simulink model "hybrid_new_eq_circuit_pascal5_single_shot_stack"  (R2019a)
settings: Solver=FixedStepAuto  StartTime=0.0  StopTime=sim_time  FixedStep=resolution  MinStep=0.001  RelTol=1e-4  EnableMultiTasking=on
values from neighbouring files (symbols this model uses):
  amps_in = double(amps_in)    [ClassHybrid.m]    (also in Sc.m = double(amps_in_); workspace_test_model.mat = 0)
  resolution = double(resolution)    [ClassHybrid.m]    (also in Sc.m = double(resolution_); matlab.mat = 1; model_out_all.mat = 0.5; testHyb.m = 0.5)
  tStep = resolution    (= 0.1)    [ClassHybrid.m]    (also in Sc.m; matlab.mat = 10; model_out_all.mat = 1; raw.mat = 1)
libraries: powerlib x525, simulink x9
(part 3 of 8)

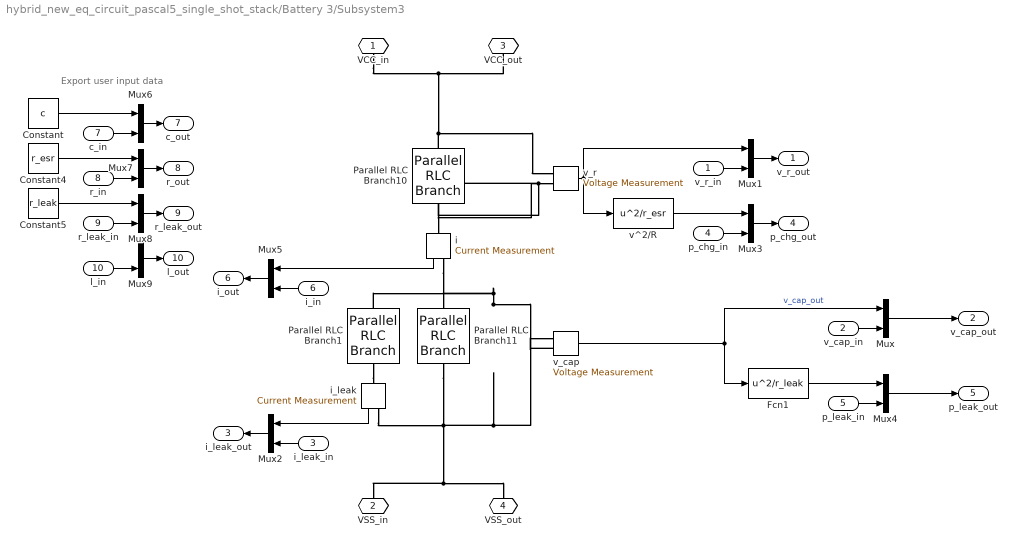
== system hybrid_new_eq_circuit_pascal5_single_shot_stack/Battery 3/Subsystem3 ==
  note: Export user input data
  v_r_in : Inport
  v_cap_in : Inport  Port=2
  i_leak_in : Inport  Port=3
  p_chg_in : Inport  Port=4
  p_leak_in : Inport  Port=5
  i_in : Inport  Port=6
  c_in : Inport  Port=7
  r_in : Inport  Port=8
  r_leak_in : Inport  Port=9
  l_in : Inport  Port=10
  Constant : Constant  Value=c
  Constant4 : Constant  Value=r_esr
  Constant5 : Constant  Value=r_leak
  Fcn1 : Fcn  Expr=u^2/r_leak
  Mux{,1..9} (10 alike) : Mux  Inputs=2
  Parallel RLC Branch1 : powerlib/Elements/Parallel RLC Branch  LConnTagsString=a  RConnTagsString=__new0  BranchType=R  Resistance=r_esr  Inductance=1e-3  SetiL0=off  InitialCurrent=0  Capacitance=1e-6  Setx0=off  InitialVoltage=0  Measurements=None
      settings: SourceProductName=Simscape Electrical
  Parallel RLC Branch10 : powerlib/Elements/Parallel RLC Branch  LConnTagsString=a  RConnTagsString=__new0  BranchType=R  Resistance=0.000001  Inductance=1e-3  SetiL0=off  InitialCurrent=0  Capacitance=1e-6  Setx0=off  InitialVoltage=0  Measurements=None
      settings: SourceProductName=Simscape Electrical
  Parallel RLC Branch11 : powerlib/Elements/Parallel RLC Branch  LConnTagsString=a  RConnTagsString=__new0  BranchType=C  Resistance=1  Inductance=1e-3  SetiL0=off  InitialCurrent=0  Capacitance=c  Setx0=on  InitialVoltage=v_init  Measurements=None
      settings: SourceProductName=Simscape Electrical
  i : powerlib/Measurements/Current Measurement  PhasorSimulation=off  OutputType=Complex  PSBequivalent=0
      settings: SourceProductName=Simscape Electrical
  i_leak : powerlib/Measurements/Current Measurement  PhasorSimulation=off  OutputType=Complex  PSBequivalent=0
      settings: SourceProductName=Simscape Electrical
  v^2/R : Fcn  Expr=u^2/r_esr
  v_cap : powerlib/Measurements/Voltage Measurement  PhasorSimulation=off  OutputType=Magnitude  PSBequivalent=0
      settings: SourceProductName=Simscape Electrical
  v_r : powerlib/Measurements/Voltage Measurement  PhasorSimulation=off  OutputType=Complex  PSBequivalent=0
      settings: SourceProductName=Simscape Electrical
  VCC_in : PMIOPort  Side=Left
  VSS_in : PMIOPort  Port=2  Side=Left
  VCC_out : PMIOPort  Tag=PMCPort  Port=3  Side=Right
  VSS_out : PMIOPort  Tag=PMCPort  Port=4  Side=Right
  v_r_out : Outport
  v_cap_out : Outport  Port=2
  i_leak_out : Outport  Port=3
  p_chg_out : Outport  Port=4
  p_leak_out : Outport  Port=5
  i_out : Outport  Port=6
  c_out : Outport  Port=7
  r_out : Outport  Port=8
  r_leak_out : Outport  Port=9
  l_out : Outport  Port=10
  wires:
  i_leak/1 -> Mux2/1
  v_r/1 -> Mux1/1, v^2/R/1
  Mux6/1 -> c_out/1
  Mux7/1 -> r_out/1
  Mux8/1 -> r_leak_out/1
  Mux9/1 -> l_out/1
  Constant/1 -> Mux6/1
  Constant4/1 -> Mux7/1
  Constant5/1 -> Mux8/1
  ? -> Mux9/1
  c_in/1 -> Mux6/2
  l_in/1 -> Mux9/2
  r_leak_in/1 -> Mux8/2
  r_in/1 -> Mux7/2
  p_chg_in/1 -> Mux3/2
  Mux3/1 -> p_chg_out/1
  v_r_in/1 -> Mux1/2
  Mux1/1 -> v_r_out/1
  v^2/R/1 -> Mux3/1
  Mux2/1 -> i_leak_out/1
  i_leak_in/1 -> Mux2/2
  i/1 -> Mux5/1
  Mux5/1 -> i_out/1
  i_in/1 -> Mux5/2
  p_leak_in/1 -> Mux4/2
  Mux4/1 -> p_leak_out/1
  Mux/1 -> v_cap_out/1
  v_cap_in/1 -> Mux/2
  Fcn1/1 -> Mux4/1
  v_cap/1 -> Fcn1/1, Mux/1  "v_cap_out"
  connections:
  VCC_in/RConn1 -- VCC_out/RConn1 -- v_r/LConn1 -- Parallel RLC Branch10/LConn1
  Parallel RLC Branch1/RConn1 -- i_leak/LConn1
  VSS_out/RConn1 -- VSS_in/RConn1 -- i_leak/RConn1 -- Parallel RLC Branch11/RConn1 -- v_cap/LConn2
  Parallel RLC Branch1/LConn1 -- i/RConn1 -- Parallel RLC Branch11/LConn1 -- v_cap/LConn1
  v_r/LConn2 -- Parallel RLC Branch10/RConn1 -- i/LConn1

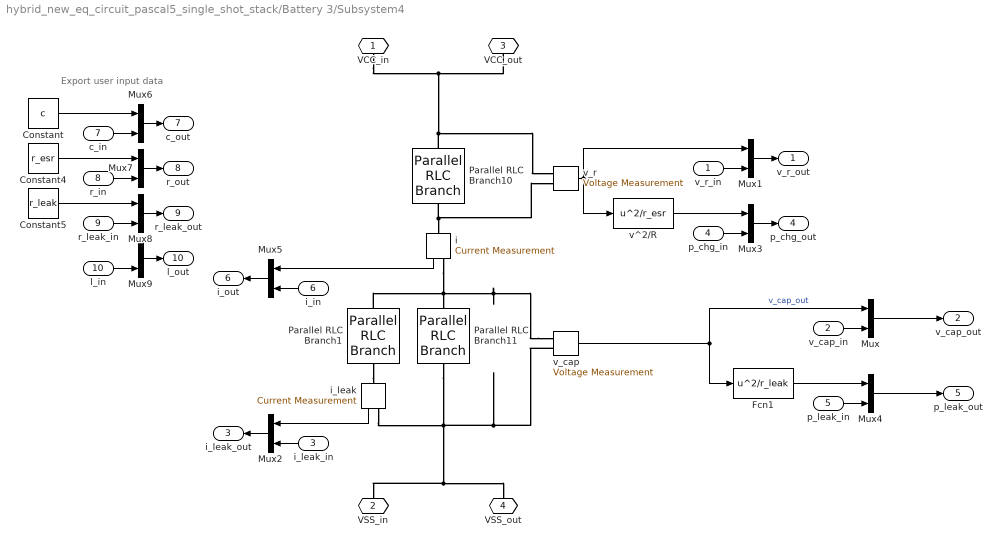
== system hybrid_new_eq_circuit_pascal5_single_shot_stack/Battery 3/Subsystem4 ==
  note: Export user input data
  v_r_in : Inport
  v_cap_in : Inport  Port=2
  i_leak_in : Inport  Port=3
  p_chg_in : Inport  Port=4
  p_leak_in : Inport  Port=5
  i_in : Inport  Port=6
  c_in : Inport  Port=7
  r_in : Inport  Port=8
  r_leak_in : Inport  Port=9
  l_in : Inport  Port=10
  Constant : Constant  Value=c
  Constant4 : Constant  Value=r_esr
  Constant5 : Constant  Value=r_leak
  Fcn1 : Fcn  Expr=u^2/r_leak
  Mux{,1..9} (10 alike) : Mux  Inputs=2
  Parallel RLC Branch1 : powerlib/Elements/Parallel RLC Branch  LConnTagsString=a  RConnTagsString=__new0  BranchType=R  Resistance=r_esr  Inductance=1e-3  SetiL0=off  InitialCurrent=0  Capacitance=1e-6  Setx0=off  InitialVoltage=0  Measurements=None
      settings: SourceProductName=Simscape Electrical
  Parallel RLC Branch10 : powerlib/Elements/Parallel RLC Branch  LConnTagsString=a  RConnTagsString=__new0  BranchType=R  Resistance=0.000001  Inductance=1e-3  SetiL0=off  InitialCurrent=0  Capacitance=1e-6  Setx0=off  InitialVoltage=0  Measurements=None
      settings: SourceProductName=Simscape Electrical
  Parallel RLC Branch11 : powerlib/Elements/Parallel RLC Branch  LConnTagsString=a  RConnTagsString=__new0  BranchType=C  Resistance=1  Inductance=1e-3  SetiL0=off  InitialCurrent=0  Capacitance=c  Setx0=on  InitialVoltage=v_init  Measurements=None
      settings: SourceProductName=Simscape Electrical
  i : powerlib/Measurements/Current Measurement  PhasorSimulation=off  OutputType=Complex  PSBequivalent=0
      settings: SourceProductName=Simscape Electrical
  i_leak : powerlib/Measurements/Current Measurement  PhasorSimulation=off  OutputType=Complex  PSBequivalent=0
      settings: SourceProductName=Simscape Electrical
  v^2/R : Fcn  Expr=u^2/r_esr
  v_cap : powerlib/Measurements/Voltage Measurement  PhasorSimulation=off  OutputType=Magnitude  PSBequivalent=0
      settings: SourceProductName=Simscape Electrical
  v_r : powerlib/Measurements/Voltage Measurement  PhasorSimulation=off  OutputType=Complex  PSBequivalent=0
      settings: SourceProductName=Simscape Electrical
  VCC_in : PMIOPort  Side=Left
  VSS_in : PMIOPort  Port=2  Side=Left
  VCC_out : PMIOPort  Tag=PMCPort  Port=3  Side=Right
  VSS_out : PMIOPort  Tag=PMCPort  Port=4  Side=Right
  v_r_out : Outport
  v_cap_out : Outport  Port=2
  i_leak_out : Outport  Port=3
  p_chg_out : Outport  Port=4
  p_leak_out : Outport  Port=5
  i_out : Outport  Port=6
  c_out : Outport  Port=7
  r_out : Outport  Port=8
  r_leak_out : Outport  Port=9
  l_out : Outport  Port=10
  wires:
  Fcn1/1 -> Mux4/1
  v_cap_in/1 -> Mux/2
  Mux/1 -> v_cap_out/1
  Mux4/1 -> p_leak_out/1
  p_leak_in/1 -> Mux4/2
  i_in/1 -> Mux5/2
  Mux5/1 -> i_out/1
  i/1 -> Mux5/1
  i_leak_in/1 -> Mux2/2
  Mux2/1 -> i_leak_out/1
  v^2/R/1 -> Mux3/1
  Mux1/1 -> v_r_out/1
  v_r_in/1 -> Mux1/2
  Mux3/1 -> p_chg_out/1
  p_chg_in/1 -> Mux3/2
  r_in/1 -> Mux7/2
  r_leak_in/1 -> Mux8/2
  l_in/1 -> Mux9/2
  c_in/1 -> Mux6/2
  ? -> Mux9/1
  Constant5/1 -> Mux8/1
  Constant4/1 -> Mux7/1
  Constant/1 -> Mux6/1
  Mux9/1 -> l_out/1
  Mux8/1 -> r_leak_out/1
  Mux7/1 -> r_out/1
  Mux6/1 -> c_out/1
  v_r/1 -> v^2/R/1, Mux1/1
  i_leak/1 -> Mux2/1
  v_cap/1 -> Mux/1, Fcn1/1  "v_cap_out"
  connections:
  i/LConn1 -- Parallel RLC Branch10/RConn1 -- v_r/LConn2
  Parallel RLC Branch10/LConn1 -- VCC_in/RConn1 -- VCC_out/RConn1 -- v_r/LConn1
  v_cap/LConn1 -- Parallel RLC Branch11/LConn1 -- i/RConn1 -- Parallel RLC Branch1/LConn1
  v_cap/LConn2 -- Parallel RLC Branch11/RConn1 -- i_leak/RConn1 -- VSS_in/RConn1 -- VSS_out/RConn1
  Parallel RLC Branch1/RConn1 -- i_leak/LConn1

== system hybrid_new_eq_circuit_pascal5_single_shot_stack/Battery 3/Subsystem8 ==
  note: Export user input data
  Constant : Constant  Value=c
  Constant4 : Constant  Value=r_esr
  Constant5 : Constant  Value=r_leak
  Fcn1 : Fcn  Expr=u^2/r_leak
  Parallel RLC Branch1 : powerlib/Elements/Parallel RLC Branch  LConnTagsString=a  RConnTagsString=__new0  BranchType=R  Resistance=r_leak  Inductance=1e-3  SetiL0=off  InitialCurrent=0  Capacitance=1e-6  Setx0=off  InitialVoltage=0  Measurements=None
      settings: SourceProductName=Simscape Electrical
  Parallel RLC Branch10 : powerlib/Elements/Parallel RLC Branch  LConnTagsString=a  RConnTagsString=__new0  BranchType=R  Resistance=0.000001  Inductance=1e-3  SetiL0=off  InitialCurrent=0  Capacitance=1e-6  Setx0=off  InitialVoltage=0  Measurements=None
      settings: SourceProductName=Simscape Electrical
  Parallel RLC Branch11 : powerlib/Elements/Parallel RLC Branch  LConnTagsString=a  RConnTagsString=__new0  BranchType=C  Resistance=1  Inductance=1e-3  SetiL0=off  InitialCurrent=0  Capacitance=c  Setx0=on  InitialVoltage=v_init  Measurements=None
      settings: SourceProductName=Simscape Electrical
  i : powerlib/Measurements/Current Measurement  PhasorSimulation=off  OutputType=Complex  PSBequivalent=0
      settings: SourceProductName=Simscape Electrical
  i_leak : powerlib/Measurements/Current Measurement  PhasorSimulation=off  OutputType=Complex  PSBequivalent=0
      settings: SourceProductName=Simscape Electrical
  v^2/R : Fcn  Expr=u^2/r_esr
  v_cap : powerlib/Measurements/Voltage Measurement  PhasorSimulation=off  OutputType=Magnitude  PSBequivalent=0
      settings: SourceProductName=Simscape Electrical
  v_r : powerlib/Measurements/Voltage Measurement  PhasorSimulation=off  OutputType=Complex  PSBequivalent=0
      settings: SourceProductName=Simscape Electrical
  VCC_in : PMIOPort  Side=Left
  VSS_in : PMIOPort  Port=2  Side=Left
  VCC_out : PMIOPort  Tag=PMCPort  Port=3  Side=Right
  VSS_out : PMIOPort  Tag=PMCPort  Port=4  Side=Right
  v_r_out : Outport
  v_cap_out : Outport  Port=2
  i_leak_out : Outport  Port=3
  p_chg_out : Outport  Port=4
  p_leak_out : Outport  Port=5
  i_out : Outport  Port=6
  c_out : Outport  Port=7
  r_out : Outport  Port=8
  r_leak_out : Outport  Port=9
  l_out : Outport  Port=10
  wires:
  v^2/R/1 -> p_chg_out/1
  Fcn1/1 -> p_leak_out/1
  v_cap/1 -> Fcn1/1, v_cap_out/1  "v_cap_out"
  i/1 -> i_out/1
  ? -> l_out/1
  Constant5/1 -> r_leak_out/1
  Constant4/1 -> r_out/1
  Constant/1 -> c_out/1
  v_r/1 -> v^2/R/1, v_r_out/1
  i_leak/1 -> i_leak_out/1
  connections:
  v_r/LConn2 -- Parallel RLC Branch10/RConn1 -- i/LConn1
  Parallel RLC Branch1/RConn1 -- i_leak/LConn1
  Parallel RLC Branch10/LConn1 -- v_r/LConn1 -- VCC_out/RConn1 -- VCC_in/RConn1
  i/RConn1 -- Parallel RLC Branch1/LConn1 -- v_cap/LConn1 -- Parallel RLC Branch11/LConn1
  i_leak/RConn1 -- v_cap/LConn2 -- VSS_in/RConn1 -- VSS_out/RConn1 -- Parallel RLC Branch11/RConn1

== system hybrid_new_eq_circuit_pascal5_single_shot_stack/Supercapacitor 1/Subsystem ==
  In1 : Inport
  In2 : Inport  Port=2
  In3 : Inport  Port=3
  In4 : Inport  Port=4
  In5 : Inport  Port=5
  In6 : Inport  Port=6
  In7 : Inport  Port=7
  In8 : Inport  Port=8
  In9 : Inport  Port=9
  In10 : Inport  Port=10
  Subsystem1 : Subsystem  mask{c=c, r_esr=r_esr, r_leak=r_leak, v_init=v_init}
      mask prompts: c "Capacitance /F"; r_esr "Series resistance /ohm"; r_leak "Leakage resistance /ohm (inf for disabled)"; v_init "Initial capacitor voltage"
  Subsystem2 : Subsystem  mask{c=c, r_esr=r_esr, r_leak=r_leak, v_init=v_init}
      mask prompts: c "Capacitance /F"; r_esr "Series resistance /ohm"; r_leak "Leakage resistance /ohm (inf for disabled)"; v_init "Initial capacitor voltage"
  Subsystem3 : Subsystem  mask{c=c, r_esr=r_esr, r_leak=r_leak, v_init=v_init}
      mask prompts: c "Capacitance /F"; r_esr "Series resistance /ohm"; r_leak "Leakage resistance /ohm (inf for disabled)"; v_init "Initial capacitor voltage"
  Subsystem5 : Subsystem  mask{c=c, r_esr=r_esr, r_leak=r_leak, v_init=v_init}
      mask prompts: c "Capacitance /F"; r_esr "Series resistance /ohm"; r_leak "Leakage resistance /ohm (inf for disabled)"; v_init "Initial capacitor voltage"
  Conn1 : PMIOPort  Side=Left
  Conn2 : PMIOPort  Port=2  Side=Right
  Conn3 : PMIOPort  Port=3  Side=Left
  Conn4 : PMIOPort  Port=4  Side=Right
  Out1 : Outport
  Out2 : Outport  Port=2
  Out3 : Outport  Port=3
  Out4 : Outport  Port=4
  Out5 : Outport  Port=5
  Out6 : Outport  Port=6
  Out7 : Outport  Port=7
  Out8 : Outport  Port=8
  Out9 : Outport  Port=9
  Out10 : Outport  Port=10
  wires:
  In8/1 -> Subsystem5/8(r_in)
  In3/1 -> Subsystem5/3(i_leak_in)
  In10/1 -> Subsystem5/10(l_in)
  In1/1 -> Subsystem5/1(v_r_in)
  In7/1 -> Subsystem5/7(c_in)
  In4/1 -> Subsystem5/4(p_chg_in)
  In5/1 -> Subsystem5/5(p_leak_in)
  In6/1 -> Subsystem5/6(i_in)
  In9/1 -> Subsystem5/9(r_leak_in)
  In2/1 -> Subsystem5/2(v_cap_in)
  Subsystem5/1(v_r_out) -> Subsystem1/1(v_r_in)
  Subsystem5/2(v_cap_out) -> Subsystem1/2(v_cap_in)
  Subsystem5/3(i_leak_out) -> Subsystem1/3(i_leak_in)
  Subsystem5/4(p_chg_out) -> Subsystem1/4(p_chg_in)
  Subsystem5/5(p_leak_out) -> Subsystem1/5(p_leak_in)
  Subsystem5/6(i_out) -> Subsystem1/6(i_in)
  Subsystem5/7(c_out) -> Subsystem1/7(c_in)
  Subsystem5/8(r_out) -> Subsystem1/8(r_in)
  Subsystem5/9(r_leak_out) -> Subsystem1/9(r_leak_in)
  Subsystem5/10(l_out) -> Subsystem1/10(l_in)
  Subsystem1/1(v_r_out) -> Subsystem2/1(v_r_in)
  Subsystem1/2(v_cap_out) -> Subsystem2/2(v_cap_in)
  Subsystem1/3(i_leak_out) -> Subsystem2/3(i_leak_in)
  Subsystem1/4(p_chg_out) -> Subsystem2/4(p_chg_in)
  Subsystem1/5(p_leak_out) -> Subsystem2/5(p_leak_in)
  Subsystem1/6(i_out) -> Subsystem2/6(i_in)
  Subsystem1/7(c_out) -> Subsystem2/7(c_in)
  Subsystem1/8(r_out) -> Subsystem2/8(r_in)
  Subsystem1/9(r_leak_out) -> Subsystem2/9(r_leak_in)
  Subsystem1/10(l_out) -> Subsystem2/10(l_in)
  Subsystem2/1(v_r_out) -> Subsystem3/1(v_r_in)
  Subsystem3/1(v_r_out) -> Out1/1
  Subsystem2/2(v_cap_out) -> Subsystem3/2(v_cap_in)
  Subsystem2/3(i_leak_out) -> Subsystem3/3(i_leak_in)
  Subsystem2/4(p_chg_out) -> Subsystem3/4(p_chg_in)
  Subsystem2/5(p_leak_out) -> Subsystem3/5(p_leak_in)
  Subsystem2/6(i_out) -> Subsystem3/6(i_in)
  Subsystem2/7(c_out) -> Subsystem3/7(c_in)
  Subsystem2/8(r_out) -> Subsystem3/8(r_in)
  Subsystem2/9(r_leak_out) -> Subsystem3/9(r_leak_in)
  Subsystem2/10(l_out) -> Subsystem3/10(l_in)
  Subsystem3/2(v_cap_out) -> Out2/1
  Subsystem3/3(i_leak_out) -> Out3/1
  Subsystem3/4(p_chg_out) -> Out4/1
  Subsystem3/5(p_leak_out) -> Out5/1
  Subsystem3/6(i_out) -> Out6/1
  Subsystem3/7(c_out) -> Out7/1
  Subsystem3/8(r_out) -> Out8/1
  Subsystem3/9(r_leak_out) -> Out9/1
  Subsystem3/10(l_out) -> Out10/1
  connections:
  Subsystem5/LConn2 -- Conn3/RConn1
  Subsystem5/LConn1 -- Conn1/RConn1
  Subsystem1/LConn1 -- Subsystem5/RConn1
  Subsystem1/LConn2 -- Subsystem5/RConn2
  Subsystem2/LConn1 -- Subsystem1/RConn1
  Subsystem2/LConn2 -- Subsystem1/RConn2
  Subsystem3/LConn1 -- Subsystem2/RConn1
  Subsystem3/LConn2 -- Subsystem2/RConn2
  Subsystem3/RConn1 -- Conn2/RConn1
  Subsystem3/RConn2 -- Conn4/RConn1

== system hybrid_new_eq_circuit_pascal5_single_shot_stack/Supercapacitor 1/Subsystem1 ==
  In1 : Inport
  In2 : Inport  Port=2
  In3 : Inport  Port=3
  In4 : Inport  Port=4
  In5 : Inport  Port=5
  In6 : Inport  Port=6
  In7 : Inport  Port=7
  In8 : Inport  Port=8
  In9 : Inport  Port=9
  In10 : Inport  Port=10
  Subsystem1 : Subsystem  mask{c=c, r_esr=r_esr, r_leak=r_leak, v_init=v_init}
      mask prompts: c "Capacitance /F"; r_esr "Series resistance /ohm"; r_leak "Leakage resistance /ohm (inf for disabled)"; v_init "Initial capacitor voltage"
  Subsystem2 : Subsystem  mask{c=c, r_esr=r_esr, r_leak=r_leak, v_init=v_init}
      mask prompts: c "Capacitance /F"; r_esr "Series resistance /ohm"; r_leak "Leakage resistance /ohm (inf for disabled)"; v_init "Initial capacitor voltage"
  Subsystem3 : Subsystem  mask{c=c, r_esr=r_esr, r_leak=r_leak, v_init=v_init}
      mask prompts: c "Capacitance /F"; r_esr "Series resistance /ohm"; r_leak "Leakage resistance /ohm (inf for disabled)"; v_init "Initial capacitor voltage"
  Subsystem5 : Subsystem  mask{c=c, r_esr=r_esr, r_leak=r_leak, v_init=v_init}
      mask prompts: c "Capacitance /F"; r_esr "Series resistance /ohm"; r_leak "Leakage resistance /ohm (inf for disabled)"; v_init "Initial capacitor voltage"
  Conn1 : PMIOPort  Side=Left
  Conn2 : PMIOPort  Port=2  Side=Right
  Conn3 : PMIOPort  Port=3  Side=Left
  Conn4 : PMIOPort  Port=4  Side=Right
  Out1 : Outport
  Out2 : Outport  Port=2
  Out3 : Outport  Port=3
  Out4 : Outport  Port=4
  Out5 : Outport  Port=5
  Out6 : Outport  Port=6
  Out7 : Outport  Port=7
  Out8 : Outport  Port=8
  Out9 : Outport  Port=9
  Out10 : Outport  Port=10
  wires:
  Subsystem3/10(l_out) -> Out10/1
  Subsystem3/9(r_leak_out) -> Out9/1
  Subsystem3/8(r_out) -> Out8/1
  Subsystem3/7(c_out) -> Out7/1
  Subsystem3/6(i_out) -> Out6/1
  Subsystem3/5(p_leak_out) -> Out5/1
  Subsystem3/4(p_chg_out) -> Out4/1
  Subsystem3/3(i_leak_out) -> Out3/1
  Subsystem3/2(v_cap_out) -> Out2/1
  Subsystem2/10(l_out) -> Subsystem3/10(l_in)
  Subsystem2/9(r_leak_out) -> Subsystem3/9(r_leak_in)
  Subsystem2/8(r_out) -> Subsystem3/8(r_in)
  Subsystem2/7(c_out) -> Subsystem3/7(c_in)
  Subsystem2/6(i_out) -> Subsystem3/6(i_in)
  Subsystem2/5(p_leak_out) -> Subsystem3/5(p_leak_in)
  Subsystem2/4(p_chg_out) -> Subsystem3/4(p_chg_in)
  Subsystem2/3(i_leak_out) -> Subsystem3/3(i_leak_in)
  Subsystem2/2(v_cap_out) -> Subsystem3/2(v_cap_in)
  Subsystem3/1(v_r_out) -> Out1/1
  Subsystem2/1(v_r_out) -> Subsystem3/1(v_r_in)
  Subsystem1/10(l_out) -> Subsystem2/10(l_in)
  Subsystem1/9(r_leak_out) -> Subsystem2/9(r_leak_in)
  Subsystem1/8(r_out) -> Subsystem2/8(r_in)
  Subsystem1/7(c_out) -> Subsystem2/7(c_in)
  Subsystem1/6(i_out) -> Subsystem2/6(i_in)
  Subsystem1/5(p_leak_out) -> Subsystem2/5(p_leak_in)
  Subsystem1/4(p_chg_out) -> Subsystem2/4(p_chg_in)
  Subsystem1/3(i_leak_out) -> Subsystem2/3(i_leak_in)
  Subsystem1/2(v_cap_out) -> Subsystem2/2(v_cap_in)
  Subsystem1/1(v_r_out) -> Subsystem2/1(v_r_in)
  Subsystem5/10(l_out) -> Subsystem1/10(l_in)
  Subsystem5/9(r_leak_out) -> Subsystem1/9(r_leak_in)
  Subsystem5/8(r_out) -> Subsystem1/8(r_in)
  Subsystem5/7(c_out) -> Subsystem1/7(c_in)
  Subsystem5/6(i_out) -> Subsystem1/6(i_in)
  Subsystem5/5(p_leak_out) -> Subsystem1/5(p_leak_in)
  Subsystem5/4(p_chg_out) -> Subsystem1/4(p_chg_in)
  Subsystem5/3(i_leak_out) -> Subsystem1/3(i_leak_in)
  Subsystem5/2(v_cap_out) -> Subsystem1/2(v_cap_in)
  Subsystem5/1(v_r_out) -> Subsystem1/1(v_r_in)
  In2/1 -> Subsystem5/2(v_cap_in)
  In9/1 -> Subsystem5/9(r_leak_in)
  In6/1 -> Subsystem5/6(i_in)
  In5/1 -> Subsystem5/5(p_leak_in)
  In4/1 -> Subsystem5/4(p_chg_in)
  In7/1 -> Subsystem5/7(c_in)
  In1/1 -> Subsystem5/1(v_r_in)
  In10/1 -> Subsystem5/10(l_in)
  In3/1 -> Subsystem5/3(i_leak_in)
  In8/1 -> Subsystem5/8(r_in)
  connections:
  Subsystem3/RConn2 -- Conn4/RConn1
  Subsystem3/RConn1 -- Conn2/RConn1
  Subsystem3/LConn2 -- Subsystem2/RConn2
  Subsystem3/LConn1 -- Subsystem2/RConn1
  Subsystem2/LConn2 -- Subsystem1/RConn2
  Subsystem2/LConn1 -- Subsystem1/RConn1
  Subsystem1/LConn2 -- Subsystem5/RConn2
  Subsystem1/LConn1 -- Subsystem5/RConn1
  Subsystem5/LConn1 -- Conn1/RConn1
  Subsystem5/LConn2 -- Conn3/RConn1

== system hybrid_new_eq_circuit_pascal5_single_shot_stack/Supercapacitor 1/Subsystem2 ==
  In1 : Inport
  In2 : Inport  Port=2
  In3 : Inport  Port=3
  In4 : Inport  Port=4
  In5 : Inport  Port=5
  In6 : Inport  Port=6
  In7 : Inport  Port=7
  In8 : Inport  Port=8
  In9 : Inport  Port=9
  In10 : Inport  Port=10
  Subsystem1 : Subsystem  mask{c=c, r_esr=r_esr, r_leak=r_leak, v_init=v_init}
      mask prompts: c "Capacitance /F"; r_esr "Series resistance /ohm"; r_leak "Leakage resistance /ohm (inf for disabled)"; v_init "Initial capacitor voltage"
  Subsystem2 : Subsystem  mask{c=c, r_esr=r_esr, r_leak=r_leak, v_init=v_init}
      mask prompts: c "Capacitance /F"; r_esr "Series resistance /ohm"; r_leak "Leakage resistance /ohm (inf for disabled)"; v_init "Initial capacitor voltage"
  Subsystem3 : Subsystem  mask{c=c, r_esr=r_esr, r_leak=r_leak, v_init=v_init}
      mask prompts: c "Capacitance /F"; r_esr "Series resistance /ohm"; r_leak "Leakage resistance /ohm (inf for disabled)"; v_init "Initial capacitor voltage"
  Subsystem4 : Subsystem  mask{c=c, r_esr=r_esr, r_leak=r_leak, v_init=v_init}
      mask prompts: c "Capacitance /F"; r_esr "Series resistance /ohm"; r_leak "Leakage resistance /ohm (inf for disabled)"; v_init "Initial capacitor voltage"
  Subsystem5 : Subsystem  mask{c=c, r_esr=r_esr, r_leak=r_leak, v_init=v_init}
      mask prompts: c "Capacitance /F"; r_esr "Series resistance /ohm"; r_leak "Leakage resistance /ohm (inf for disabled)"; v_init "Initial capacitor voltage"
  Subsystem6 : Subsystem  mask{c=c, r_esr=r_esr, r_leak=r_leak, v_init=v_init}
      mask prompts: c "Capacitance /F"; r_esr "Series resistance /ohm"; r_leak "Leakage resistance /ohm (inf for disabled)"; v_init "Initial capacitor voltage"
  Conn1 : PMIOPort  Side=Left
  Conn2 : PMIOPort  Port=2  Side=Right
  Conn3 : PMIOPort  Port=3  Side=Left
  Conn4 : PMIOPort  Port=4  Side=Right
  Out1 : Outport
  Out2 : Outport  Port=2
  Out3 : Outport  Port=3
  Out4 : Outport  Port=4
  Out5 : Outport  Port=5
  Out6 : Outport  Port=6
  Out7 : Outport  Port=7
  Out8 : Outport  Port=8
  Out9 : Outport  Port=9
  Out10 : Outport  Port=10
  wires:
  In1/1 -> Subsystem5/1(v_r_in)
  In2/1 -> Subsystem5/2(v_cap_in)
  In3/1 -> Subsystem5/3(i_leak_in)
  In4/1 -> Subsystem5/4(p_chg_in)
  In5/1 -> Subsystem5/5(p_leak_in)
  In6/1 -> Subsystem5/6(i_in)
  In7/1 -> Subsystem5/7(c_in)
  In8/1 -> Subsystem5/8(r_in)
  In9/1 -> Subsystem5/9(r_leak_in)
  In10/1 -> Subsystem5/10(l_in)
  Subsystem5/1(v_r_out) -> Subsystem1/1(v_r_in)
  Subsystem5/2(v_cap_out) -> Subsystem1/2(v_cap_in)
  Subsystem5/3(i_leak_out) -> Subsystem1/3(i_leak_in)
  Subsystem5/4(p_chg_out) -> Subsystem1/4(p_chg_in)
  Subsystem5/5(p_leak_out) -> Subsystem1/5(p_leak_in)
  Subsystem5/6(i_out) -> Subsystem1/6(i_in)
  Subsystem5/7(c_out) -> Subsystem1/7(c_in)
  Subsystem5/8(r_out) -> Subsystem1/8(r_in)
  Subsystem5/9(r_leak_out) -> Subsystem1/9(r_leak_in)
  Subsystem5/10(l_out) -> Subsystem1/10(l_in)
  Subsystem1/1(v_r_out) -> Subsystem2/1(v_r_in)
  Subsystem1/2(v_cap_out) -> Subsystem2/2(v_cap_in)
  Subsystem1/3(i_leak_out) -> Subsystem2/3(i_leak_in)
  Subsystem1/4(p_chg_out) -> Subsystem2/4(p_chg_in)
  Subsystem1/5(p_leak_out) -> Subsystem2/5(p_leak_in)
  Subsystem1/6(i_out) -> Subsystem2/6(i_in)
  Subsystem1/7(c_out) -> Subsystem2/7(c_in)
  Subsystem1/8(r_out) -> Subsystem2/8(r_in)
  Subsystem1/9(r_leak_out) -> Subsystem2/9(r_leak_in)
  Subsystem1/10(l_out) -> Subsystem2/10(l_in)
  Subsystem2/1(v_r_out) -> Subsystem3/1(v_r_in)
  Subsystem2/2(v_cap_out) -> Subsystem3/2(v_cap_in)
  Subsystem2/3(i_leak_out) -> Subsystem3/3(i_leak_in)
  Subsystem2/4(p_chg_out) -> Subsystem3/4(p_chg_in)
  Subsystem2/5(p_leak_out) -> Subsystem3/5(p_leak_in)
  Subsystem2/6(i_out) -> Subsystem3/6(i_in)
  Subsystem2/7(c_out) -> Subsystem3/7(c_in)
  Subsystem2/8(r_out) -> Subsystem3/8(r_in)
  Subsystem2/9(r_leak_out) -> Subsystem3/9(r_leak_in)
  Subsystem2/10(l_out) -> Subsystem3/10(l_in)
  Subsystem3/1(v_r_out) -> Subsystem4/1(v_r_in)
  Subsystem3/2(v_cap_out) -> Subsystem4/2(v_cap_in)
  Subsystem3/3(i_leak_out) -> Subsystem4/3(i_leak_in)
  Subsystem3/4(p_chg_out) -> Subsystem4/4(p_chg_in)
  Subsystem3/5(p_leak_out) -> Subsystem4/5(p_leak_in)
  Subsystem3/6(i_out) -> Subsystem4/6(i_in)
  Subsystem3/7(c_out) -> Subsystem4/7(c_in)
  Subsystem3/8(r_out) -> Subsystem4/8(r_in)
  Subsystem3/9(r_leak_out) -> Subsystem4/9(r_leak_in)
  Subsystem3/10(l_out) -> Subsystem4/10(l_in)
  Subsystem4/1(v_r_out) -> Subsystem6/1(v_r_in)
  Subsystem4/2(v_cap_out) -> Subsystem6/2(v_cap_in)
  Subsystem4/3(i_leak_out) -> Subsystem6/3(i_leak_in)
  Subsystem4/4(p_chg_out) -> Subsystem6/4(p_chg_in)
  Subsystem4/5(p_leak_out) -> Subsystem6/5(p_leak_in)
  Subsystem4/6(i_out) -> Subsystem6/6(i_in)
  Subsystem4/7(c_out) -> Subsystem6/7(c_in)
  Subsystem4/8(r_out) -> Subsystem6/8(r_in)
  Subsystem4/9(r_leak_out) -> Subsystem6/9(r_leak_in)
  Subsystem4/10(l_out) -> Subsystem6/10(l_in)
  Subsystem6/1(v_r_out) -> Out1/1
  Subsystem6/2(v_cap_out) -> Out2/1
  Subsystem6/3(i_leak_out) -> Out3/1
  Subsystem6/4(p_chg_out) -> Out4/1
  Subsystem6/5(p_leak_out) -> Out5/1
  Subsystem6/6(i_out) -> Out6/1
  Subsystem6/7(c_out) -> Out7/1
  Subsystem6/8(r_out) -> Out8/1
  Subsystem6/9(r_leak_out) -> Out9/1
  Subsystem6/10(l_out) -> Out10/1
  connections:
  Conn1/RConn1 -- Subsystem5/LConn1
  Conn3/RConn1 -- Subsystem5/LConn2
  Subsystem1/LConn1 -- Subsystem5/RConn1
  Subsystem1/LConn2 -- Subsystem5/RConn2
  Subsystem2/LConn1 -- Subsystem1/RConn1
  Subsystem2/LConn2 -- Subsystem1/RConn2
  Subsystem3/LConn1 -- Subsystem2/RConn1
  Subsystem3/LConn2 -- Subsystem2/RConn2
  Subsystem4/LConn1 -- Subsystem3/RConn1
  Subsystem4/LConn2 -- Subsystem3/RConn2
  Subsystem6/LConn1 -- Subsystem4/RConn1
  Subsystem6/LConn2 -- Subsystem4/RConn2
  Subsystem6/RConn1 -- Conn2/RConn1
  Subsystem6/RConn2 -- Conn4/RConn1

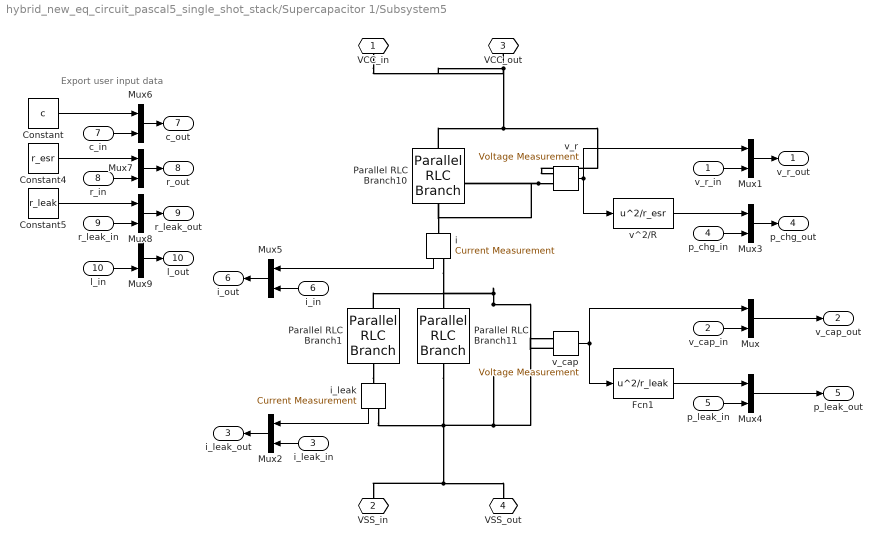
== system hybrid_new_eq_circuit_pascal5_single_shot_stack/Supercapacitor 1/Subsystem5 ==
  note: Export user input data
  v_r_in : Inport
  v_cap_in : Inport  Port=2
  i_leak_in : Inport  Port=3
  p_chg_in : Inport  Port=4
  p_leak_in : Inport  Port=5
  i_in : Inport  Port=6
  c_in : Inport  Port=7
  r_in : Inport  Port=8
  r_leak_in : Inport  Port=9
  l_in : Inport  Port=10
  Constant : Constant  Value=c
  Constant4 : Constant  Value=r_esr
  Constant5 : Constant  Value=r_leak
  Fcn1 : Fcn  Expr=u^2/r_leak
  Mux{,1..9} (10 alike) : Mux  Inputs=2
  Parallel RLC Branch1 : powerlib/Elements/Parallel RLC Branch  LConnTagsString=a  RConnTagsString=__new0  BranchType=R  Resistance=r_esr  Inductance=1e-3  SetiL0=off  InitialCurrent=0  Capacitance=1e-6  Setx0=off  InitialVoltage=0  Measurements=None
      settings: SourceProductName=Simscape Electrical
  Parallel RLC Branch10 : powerlib/Elements/Parallel RLC Branch  LConnTagsString=a  RConnTagsString=__new0  BranchType=R  Resistance=r_esr  Inductance=1e-3  SetiL0=off  InitialCurrent=0  Capacitance=1e-6  Setx0=off  InitialVoltage=0  Measurements=None
      settings: SourceProductName=Simscape Electrical
  Parallel RLC Branch11 : powerlib/Elements/Parallel RLC Branch  LConnTagsString=a  RConnTagsString=__new0  BranchType=C  Resistance=1  Inductance=1e-3  SetiL0=off  InitialCurrent=0  Capacitance=c  Setx0=on  InitialVoltage=v_init  Measurements=None
      settings: SourceProductName=Simscape Electrical
  i : powerlib/Measurements/Current Measurement  PhasorSimulation=off  OutputType=Complex  PSBequivalent=0
      settings: SourceProductName=Simscape Electrical
  i_leak : powerlib/Measurements/Current Measurement  PhasorSimulation=off  OutputType=Complex  PSBequivalent=0
      settings: SourceProductName=Simscape Electrical
  v^2/R : Fcn  Expr=u^2/r_esr
  v_cap : powerlib/Measurements/Voltage Measurement  PhasorSimulation=off  OutputType=Complex  PSBequivalent=0
      settings: SourceProductName=Simscape Electrical
  v_r : powerlib/Measurements/Voltage Measurement  PhasorSimulation=off  OutputType=Complex  PSBequivalent=0
      settings: SourceProductName=Simscape Electrical
  VCC_in : PMIOPort  Side=Left
  VSS_in : PMIOPort  Port=2  Side=Left
  VCC_out : PMIOPort  Tag=PMCPort  Port=3  Side=Right
  VSS_out : PMIOPort  Tag=PMCPort  Port=4  Side=Right
  v_r_out : Outport
  v_cap_out : Outport  Port=2
  i_leak_out : Outport  Port=3
  p_chg_out : Outport  Port=4
  p_leak_out : Outport  Port=5
  i_out : Outport  Port=6
  c_out : Outport  Port=7
  r_out : Outport  Port=8
  r_leak_out : Outport  Port=9
  l_out : Outport  Port=10
  wires:
  i_leak/1 -> Mux2/1
  v_r/1 -> Mux1/1, v^2/R/1
  Mux6/1 -> c_out/1
  Mux7/1 -> r_out/1
  Mux8/1 -> r_leak_out/1
  Mux9/1 -> l_out/1
  Constant/1 -> Mux6/1
  Constant4/1 -> Mux7/1
  Constant5/1 -> Mux8/1
  ? -> Mux9/1
  c_in/1 -> Mux6/2
  l_in/1 -> Mux9/2
  r_leak_in/1 -> Mux8/2
  r_in/1 -> Mux7/2
  p_chg_in/1 -> Mux3/2
  Mux3/1 -> p_chg_out/1
  v_r_in/1 -> Mux1/2
  Mux1/1 -> v_r_out/1
  v^2/R/1 -> Mux3/1
  Mux2/1 -> i_leak_out/1
  i_leak_in/1 -> Mux2/2
  i/1 -> Mux5/1
  Mux5/1 -> i_out/1
  i_in/1 -> Mux5/2
  p_leak_in/1 -> Mux4/2
  Mux4/1 -> p_leak_out/1
  Mux/1 -> v_cap_out/1
  v_cap_in/1 -> Mux/2
  v_cap/1 -> Fcn1/1, Mux/1
  Fcn1/1 -> Mux4/1
  connections:
  Parallel RLC Branch1/RConn1 -- i_leak/LConn1
  VSS_out/RConn1 -- VSS_in/RConn1 -- i_leak/RConn1 -- Parallel RLC Branch11/RConn1 -- v_cap/LConn2
  Parallel RLC Branch1/LConn1 -- i/RConn1 -- Parallel RLC Branch11/LConn1 -- v_cap/LConn1
  VCC_out/RConn1 -- v_r/LConn1 -- Parallel RLC Branch10/LConn1 -- VCC_in/RConn1
  v_r/LConn2 -- i/LConn1 -- Parallel RLC Branch10/RConn1

== system hybrid_new_eq_circuit_pascal5_single_shot_stack/Supercapacitor 1/Subsystem8 ==
  note: Export user input data
  Constant : Constant  Value=c
  Constant4 : Constant  Value=r_esr
  Constant5 : Constant  Value=r_leak
  Fcn1 : Fcn  Expr=u^2/r_leak
  Parallel RLC Branch1 : powerlib/Elements/Parallel RLC Branch  LConnTagsString=a  RConnTagsString=__new0  BranchType=R  Resistance=r_leak  Inductance=1e-3  SetiL0=off  InitialCurrent=0  Capacitance=1e-6  Setx0=off  InitialVoltage=0  Measurements=None
      settings: SourceProductName=Simscape Electrical
  Parallel RLC Branch10 : powerlib/Elements/Parallel RLC Branch  LConnTagsString=a  RConnTagsString=__new0  BranchType=R  Resistance=r_esr  Inductance=1e-3  SetiL0=off  InitialCurrent=0  Capacitance=1e-6  Setx0=off  InitialVoltage=0  Measurements=None
      settings: SourceProductName=Simscape Electrical
  Parallel RLC Branch11 : powerlib/Elements/Parallel RLC Branch  LConnTagsString=a  RConnTagsString=__new0  BranchType=C  Resistance=1  Inductance=1e-3  SetiL0=off  InitialCurrent=0  Capacitance=c  Setx0=on  InitialVoltage=v_init  Measurements=None
      settings: SourceProductName=Simscape Electrical
  i : powerlib/Measurements/Current Measurement  PhasorSimulation=off  OutputType=Complex  PSBequivalent=0
      settings: SourceProductName=Simscape Electrical
  i_leak : powerlib/Measurements/Current Measurement  PhasorSimulation=off  OutputType=Complex  PSBequivalent=0
      settings: SourceProductName=Simscape Electrical
  v^2/R : Fcn  Expr=u^2/r_esr
  v_cap : powerlib/Measurements/Voltage Measurement  PhasorSimulation=off  OutputType=Complex  PSBequivalent=0
      settings: SourceProductName=Simscape Electrical
  v_r : powerlib/Measurements/Voltage Measurement  PhasorSimulation=off  OutputType=Complex  PSBequivalent=0
      settings: SourceProductName=Simscape Electrical
  VCC_in : PMIOPort  Side=Left
  VSS_in : PMIOPort  Port=2  Side=Left
  VCC_out : PMIOPort  Tag=PMCPort  Port=3  Side=Right
  VSS_out : PMIOPort  Tag=PMCPort  Port=4  Side=Right
  v_r_out : Outport
  v_cap_out : Outport  Port=2
  i_leak_out : Outport  Port=3
  p_chg_out : Outport  Port=4
  p_leak_out : Outport  Port=5
  i_out : Outport  Port=6
  c_out : Outport  Port=7
  r_out : Outport  Port=8
  r_leak_out : Outport  Port=9
  l_out : Outport  Port=10
  wires:
  i_leak/1 -> i_leak_out/1
  v_r/1 -> v_r_out/1, v^2/R/1
  Constant/1 -> c_out/1
  Constant4/1 -> r_out/1
  Constant5/1 -> r_leak_out/1
  ? -> l_out/1
  i/1 -> i_out/1
  v_cap/1 -> v_cap_out/1, Fcn1/1
  Fcn1/1 -> p_leak_out/1
  v^2/R/1 -> p_chg_out/1
  connections:
  Parallel RLC Branch11/RConn1 -- v_cap/LConn2 -- i_leak/RConn1 -- VSS_out/RConn1 -- VSS_in/RConn1
  Parallel RLC Branch11/LConn1 -- Parallel RLC Branch1/LConn1 -- i/RConn1 -- v_cap/LConn1
  VCC_in/RConn1 -- VCC_out/RConn1 -- Parallel RLC Branch10/LConn1 -- v_r/LConn1
  Parallel RLC Branch10/RConn1 -- v_r/LConn2 -- i/LConn1
  Parallel RLC Branch1/RConn1 -- i_leak/LConn1

== system hybrid_new_eq_circuit_pascal5_single_shot_stack/Supercapacitor 2/Subsystem ==
  In1 : Inport
  In2 : Inport  Port=2
  In3 : Inport  Port=3
  In4 : Inport  Port=4
  In5 : Inport  Port=5
  In6 : Inport  Port=6
  In7 : Inport  Port=7
  In8 : Inport  Port=8
  In9 : Inport  Port=9
  In10 : Inport  Port=10
  Subsystem1 : Subsystem  mask{c=c, r_esr=r_esr, r_leak=r_leak, v_init=v_init}
      mask prompts: c "Capacitance /F"; r_esr "Series resistance /ohm"; r_leak "Leakage resistance /ohm (inf for disabled)"; v_init "Initial capacitor voltage"
  Subsystem2 : Subsystem  mask{c=c, r_esr=r_esr, r_leak=r_leak, v_init=v_init}
      mask prompts: c "Capacitance /F"; r_esr "Series resistance /ohm"; r_leak "Leakage resistance /ohm (inf for disabled)"; v_init "Initial capacitor voltage"
  Subsystem3 : Subsystem  mask{c=c, r_esr=r_esr, r_leak=r_leak, v_init=v_init}
      mask prompts: c "Capacitance /F"; r_esr "Series resistance /ohm"; r_leak "Leakage resistance /ohm (inf for disabled)"; v_init "Initial capacitor voltage"
  Subsystem5 : Subsystem  mask{c=c, r_esr=r_esr, r_leak=r_leak, v_init=v_init}
      mask prompts: c "Capacitance /F"; r_esr "Series resistance /ohm"; r_leak "Leakage resistance /ohm (inf for disabled)"; v_init "Initial capacitor voltage"
  Conn1 : PMIOPort  Side=Left
  Conn2 : PMIOPort  Port=2  Side=Right
  Conn3 : PMIOPort  Port=3  Side=Left
  Conn4 : PMIOPort  Port=4  Side=Right
  Out1 : Outport
  Out2 : Outport  Port=2
  Out3 : Outport  Port=3
  Out4 : Outport  Port=4
  Out5 : Outport  Port=5
  Out6 : Outport  Port=6
  Out7 : Outport  Port=7
  Out8 : Outport  Port=8
  Out9 : Outport  Port=9
  Out10 : Outport  Port=10
  wires:
  Subsystem3/10(l_out) -> Out10/1
  Subsystem3/9(r_leak_out) -> Out9/1
  Subsystem3/8(r_out) -> Out8/1
  Subsystem3/7(c_out) -> Out7/1
  Subsystem3/6(i_out) -> Out6/1
  Subsystem3/5(p_leak_out) -> Out5/1
  Subsystem3/4(p_chg_out) -> Out4/1
  Subsystem3/3(i_leak_out) -> Out3/1
  Subsystem3/2(v_cap_out) -> Out2/1
  Subsystem2/10(l_out) -> Subsystem3/10(l_in)
  Subsystem2/9(r_leak_out) -> Subsystem3/9(r_leak_in)
  Subsystem2/8(r_out) -> Subsystem3/8(r_in)
  Subsystem2/7(c_out) -> Subsystem3/7(c_in)
  Subsystem2/6(i_out) -> Subsystem3/6(i_in)
  Subsystem2/5(p_leak_out) -> Subsystem3/5(p_leak_in)
  Subsystem2/4(p_chg_out) -> Subsystem3/4(p_chg_in)
  Subsystem2/3(i_leak_out) -> Subsystem3/3(i_leak_in)
  Subsystem2/2(v_cap_out) -> Subsystem3/2(v_cap_in)
  Subsystem3/1(v_r_out) -> Out1/1
  Subsystem2/1(v_r_out) -> Subsystem3/1(v_r_in)
  Subsystem1/10(l_out) -> Subsystem2/10(l_in)
  Subsystem1/9(r_leak_out) -> Subsystem2/9(r_leak_in)
  Subsystem1/8(r_out) -> Subsystem2/8(r_in)
  Subsystem1/7(c_out) -> Subsystem2/7(c_in)
  Subsystem1/6(i_out) -> Subsystem2/6(i_in)
  Subsystem1/5(p_leak_out) -> Subsystem2/5(p_leak_in)
  Subsystem1/4(p_chg_out) -> Subsystem2/4(p_chg_in)
  Subsystem1/3(i_leak_out) -> Subsystem2/3(i_leak_in)
  Subsystem1/2(v_cap_out) -> Subsystem2/2(v_cap_in)
  Subsystem1/1(v_r_out) -> Subsystem2/1(v_r_in)
  Subsystem5/10(l_out) -> Subsystem1/10(l_in)
  Subsystem5/9(r_leak_out) -> Subsystem1/9(r_leak_in)
  Subsystem5/8(r_out) -> Subsystem1/8(r_in)
  Subsystem5/7(c_out) -> Subsystem1/7(c_in)
  Subsystem5/6(i_out) -> Subsystem1/6(i_in)
  Subsystem5/5(p_leak_out) -> Subsystem1/5(p_leak_in)
  Subsystem5/4(p_chg_out) -> Subsystem1/4(p_chg_in)
  Subsystem5/3(i_leak_out) -> Subsystem1/3(i_leak_in)
  Subsystem5/2(v_cap_out) -> Subsystem1/2(v_cap_in)
  Subsystem5/1(v_r_out) -> Subsystem1/1(v_r_in)
  In2/1 -> Subsystem5/2(v_cap_in)
  In9/1 -> Subsystem5/9(r_leak_in)
  In6/1 -> Subsystem5/6(i_in)
  In5/1 -> Subsystem5/5(p_leak_in)
  In4/1 -> Subsystem5/4(p_chg_in)
  In7/1 -> Subsystem5/7(c_in)
  In1/1 -> Subsystem5/1(v_r_in)
  In10/1 -> Subsystem5/10(l_in)
  In3/1 -> Subsystem5/3(i_leak_in)
  In8/1 -> Subsystem5/8(r_in)
  connections:
  Subsystem3/RConn2 -- Conn4/RConn1
  Subsystem3/RConn1 -- Conn2/RConn1
  Subsystem3/LConn2 -- Subsystem2/RConn2
  Subsystem3/LConn1 -- Subsystem2/RConn1
  Subsystem2/LConn2 -- Subsystem1/RConn2
  Subsystem2/LConn1 -- Subsystem1/RConn1
  Subsystem1/LConn2 -- Subsystem5/RConn2
  Subsystem1/LConn1 -- Subsystem5/RConn1
  Subsystem5/LConn1 -- Conn1/RConn1
  Subsystem5/LConn2 -- Conn3/RConn1

== system hybrid_new_eq_circuit_pascal5_single_shot_stack/Supercapacitor 2/Subsystem1 ==
  In1 : Inport
  In2 : Inport  Port=2
  In3 : Inport  Port=3
  In4 : Inport  Port=4
  In5 : Inport  Port=5
  In6 : Inport  Port=6
  In7 : Inport  Port=7
  In8 : Inport  Port=8
  In9 : Inport  Port=9
  In10 : Inport  Port=10
  Subsystem1 : Subsystem  mask{c=c, r_esr=r_esr, r_leak=r_leak, v_init=v_init}
      mask prompts: c "Capacitance /F"; r_esr "Series resistance /ohm"; r_leak "Leakage resistance /ohm (inf for disabled)"; v_init "Initial capacitor voltage"
  Subsystem2 : Subsystem  mask{c=c, r_esr=r_esr, r_leak=r_leak, v_init=v_init}
      mask prompts: c "Capacitance /F"; r_esr "Series resistance /ohm"; r_leak "Leakage resistance /ohm (inf for disabled)"; v_init "Initial capacitor voltage"
  Subsystem3 : Subsystem  mask{c=c, r_esr=r_esr, r_leak=r_leak, v_init=v_init}
      mask prompts: c "Capacitance /F"; r_esr "Series resistance /ohm"; r_leak "Leakage resistance /ohm (inf for disabled)"; v_init "Initial capacitor voltage"
  Subsystem5 : Subsystem  mask{c=c, r_esr=r_esr, r_leak=r_leak, v_init=v_init}
      mask prompts: c "Capacitance /F"; r_esr "Series resistance /ohm"; r_leak "Leakage resistance /ohm (inf for disabled)"; v_init "Initial capacitor voltage"
  Conn1 : PMIOPort  Side=Left
  Conn2 : PMIOPort  Port=2  Side=Right
  Conn3 : PMIOPort  Port=3  Side=Left
  Conn4 : PMIOPort  Port=4  Side=Right
  Out1 : Outport
  Out2 : Outport  Port=2
  Out3 : Outport  Port=3
  Out4 : Outport  Port=4
  Out5 : Outport  Port=5
  Out6 : Outport  Port=6
  Out7 : Outport  Port=7
  Out8 : Outport  Port=8
  Out9 : Outport  Port=9
  Out10 : Outport  Port=10
  wires:
  In8/1 -> Subsystem5/8(r_in)
  In3/1 -> Subsystem5/3(i_leak_in)
  In10/1 -> Subsystem5/10(l_in)
  In1/1 -> Subsystem5/1(v_r_in)
  In7/1 -> Subsystem5/7(c_in)
  In4/1 -> Subsystem5/4(p_chg_in)
  In5/1 -> Subsystem5/5(p_leak_in)
  In6/1 -> Subsystem5/6(i_in)
  In9/1 -> Subsystem5/9(r_leak_in)
  In2/1 -> Subsystem5/2(v_cap_in)
  Subsystem5/1(v_r_out) -> Subsystem1/1(v_r_in)
  Subsystem5/2(v_cap_out) -> Subsystem1/2(v_cap_in)
  Subsystem5/3(i_leak_out) -> Subsystem1/3(i_leak_in)
  Subsystem5/4(p_chg_out) -> Subsystem1/4(p_chg_in)
  Subsystem5/5(p_leak_out) -> Subsystem1/5(p_leak_in)
  Subsystem5/6(i_out) -> Subsystem1/6(i_in)
  Subsystem5/7(c_out) -> Subsystem1/7(c_in)
  Subsystem5/8(r_out) -> Subsystem1/8(r_in)
  Subsystem5/9(r_leak_out) -> Subsystem1/9(r_leak_in)
  Subsystem5/10(l_out) -> Subsystem1/10(l_in)
  Subsystem1/1(v_r_out) -> Subsystem2/1(v_r_in)
  Subsystem1/2(v_cap_out) -> Subsystem2/2(v_cap_in)
  Subsystem1/3(i_leak_out) -> Subsystem2/3(i_leak_in)
  Subsystem1/4(p_chg_out) -> Subsystem2/4(p_chg_in)
  Subsystem1/5(p_leak_out) -> Subsystem2/5(p_leak_in)
  Subsystem1/6(i_out) -> Subsystem2/6(i_in)
  Subsystem1/7(c_out) -> Subsystem2/7(c_in)
  Subsystem1/8(r_out) -> Subsystem2/8(r_in)
  Subsystem1/9(r_leak_out) -> Subsystem2/9(r_leak_in)
  Subsystem1/10(l_out) -> Subsystem2/10(l_in)
  Subsystem2/1(v_r_out) -> Subsystem3/1(v_r_in)
  Subsystem3/1(v_r_out) -> Out1/1
  Subsystem2/2(v_cap_out) -> Subsystem3/2(v_cap_in)
  Subsystem2/3(i_leak_out) -> Subsystem3/3(i_leak_in)
  Subsystem2/4(p_chg_out) -> Subsystem3/4(p_chg_in)
  Subsystem2/5(p_leak_out) -> Subsystem3/5(p_leak_in)
  Subsystem2/6(i_out) -> Subsystem3/6(i_in)
  Subsystem2/7(c_out) -> Subsystem3/7(c_in)
  Subsystem2/8(r_out) -> Subsystem3/8(r_in)
  Subsystem2/9(r_leak_out) -> Subsystem3/9(r_leak_in)
  Subsystem2/10(l_out) -> Subsystem3/10(l_in)
  Subsystem3/2(v_cap_out) -> Out2/1
  Subsystem3/3(i_leak_out) -> Out3/1
  Subsystem3/4(p_chg_out) -> Out4/1
  Subsystem3/5(p_leak_out) -> Out5/1
  Subsystem3/6(i_out) -> Out6/1
  Subsystem3/7(c_out) -> Out7/1
  Subsystem3/8(r_out) -> Out8/1
  Subsystem3/9(r_leak_out) -> Out9/1
  Subsystem3/10(l_out) -> Out10/1
  connections:
  Subsystem5/LConn2 -- Conn3/RConn1
  Subsystem5/LConn1 -- Conn1/RConn1
  Subsystem1/LConn1 -- Subsystem5/RConn1
  Subsystem1/LConn2 -- Subsystem5/RConn2
  Subsystem2/LConn1 -- Subsystem1/RConn1
  Subsystem2/LConn2 -- Subsystem1/RConn2
  Subsystem3/LConn1 -- Subsystem2/RConn1
  Subsystem3/LConn2 -- Subsystem2/RConn2
  Subsystem3/RConn1 -- Conn2/RConn1
  Subsystem3/RConn2 -- Conn4/RConn1

== system hybrid_new_eq_circuit_pascal5_single_shot_stack/Supercapacitor 2/Subsystem2 ==
  In1 : Inport
  In2 : Inport  Port=2
  In3 : Inport  Port=3
  In4 : Inport  Port=4
  In5 : Inport  Port=5
  In6 : Inport  Port=6
  In7 : Inport  Port=7
  In8 : Inport  Port=8
  In9 : Inport  Port=9
  In10 : Inport  Port=10
  Subsystem1 : Subsystem  mask{c=c, r_esr=r_esr, r_leak=r_leak, v_init=v_init}
      mask prompts: c "Capacitance /F"; r_esr "Series resistance /ohm"; r_leak "Leakage resistance /ohm (inf for disabled)"; v_init "Initial capacitor voltage"
  Subsystem2 : Subsystem  mask{c=c, r_esr=r_esr, r_leak=r_leak, v_init=v_init}
      mask prompts: c "Capacitance /F"; r_esr "Series resistance /ohm"; r_leak "Leakage resistance /ohm (inf for disabled)"; v_init "Initial capacitor voltage"
  Subsystem3 : Subsystem  mask{c=c, r_esr=r_esr, r_leak=r_leak, v_init=v_init}
      mask prompts: c "Capacitance /F"; r_esr "Series resistance /ohm"; r_leak "Leakage resistance /ohm (inf for disabled)"; v_init "Initial capacitor voltage"
  Subsystem4 : Subsystem  mask{c=c, r_esr=r_esr, r_leak=r_leak, v_init=v_init}
      mask prompts: c "Capacitance /F"; r_esr "Series resistance /ohm"; r_leak "Leakage resistance /ohm (inf for disabled)"; v_init "Initial capacitor voltage"
  Subsystem5 : Subsystem  mask{c=c, r_esr=r_esr, r_leak=r_leak, v_init=v_init}
      mask prompts: c "Capacitance /F"; r_esr "Series resistance /ohm"; r_leak "Leakage resistance /ohm (inf for disabled)"; v_init "Initial capacitor voltage"
  Subsystem6 : Subsystem  mask{c=c, r_esr=r_esr, r_leak=r_leak, v_init=v_init}
      mask prompts: c "Capacitance /F"; r_esr "Series resistance /ohm"; r_leak "Leakage resistance /ohm (inf for disabled)"; v_init "Initial capacitor voltage"
  Conn1 : PMIOPort  Side=Left
  Conn2 : PMIOPort  Port=2  Side=Right
  Conn3 : PMIOPort  Port=3  Side=Left
  Conn4 : PMIOPort  Port=4  Side=Right
  Out1 : Outport
  Out2 : Outport  Port=2
  Out3 : Outport  Port=3
  Out4 : Outport  Port=4
  Out5 : Outport  Port=5
  Out6 : Outport  Port=6
  Out7 : Outport  Port=7
  Out8 : Outport  Port=8
  Out9 : Outport  Port=9
  Out10 : Outport  Port=10
  wires:
  Subsystem6/10(l_out) -> Out10/1
  Subsystem6/9(r_leak_out) -> Out9/1
  Subsystem6/8(r_out) -> Out8/1
  Subsystem6/7(c_out) -> Out7/1
  Subsystem6/6(i_out) -> Out6/1
  Subsystem6/5(p_leak_out) -> Out5/1
  Subsystem6/4(p_chg_out) -> Out4/1
  Subsystem6/3(i_leak_out) -> Out3/1
  Subsystem6/2(v_cap_out) -> Out2/1
  Subsystem6/1(v_r_out) -> Out1/1
  Subsystem4/10(l_out) -> Subsystem6/10(l_in)
  Subsystem4/9(r_leak_out) -> Subsystem6/9(r_leak_in)
  Subsystem4/8(r_out) -> Subsystem6/8(r_in)
  Subsystem4/7(c_out) -> Subsystem6/7(c_in)
  Subsystem4/6(i_out) -> Subsystem6/6(i_in)
  Subsystem4/5(p_leak_out) -> Subsystem6/5(p_leak_in)
  Subsystem4/4(p_chg_out) -> Subsystem6/4(p_chg_in)
  Subsystem4/3(i_leak_out) -> Subsystem6/3(i_leak_in)
  Subsystem4/2(v_cap_out) -> Subsystem6/2(v_cap_in)
  Subsystem4/1(v_r_out) -> Subsystem6/1(v_r_in)
  Subsystem3/10(l_out) -> Subsystem4/10(l_in)
  Subsystem3/9(r_leak_out) -> Subsystem4/9(r_leak_in)
  Subsystem3/8(r_out) -> Subsystem4/8(r_in)
  Subsystem3/7(c_out) -> Subsystem4/7(c_in)
  Subsystem3/6(i_out) -> Subsystem4/6(i_in)
  Subsystem3/5(p_leak_out) -> Subsystem4/5(p_leak_in)
  Subsystem3/4(p_chg_out) -> Subsystem4/4(p_chg_in)
  Subsystem3/3(i_leak_out) -> Subsystem4/3(i_leak_in)
  Subsystem3/2(v_cap_out) -> Subsystem4/2(v_cap_in)
  Subsystem3/1(v_r_out) -> Subsystem4/1(v_r_in)
  Subsystem2/10(l_out) -> Subsystem3/10(l_in)
  Subsystem2/9(r_leak_out) -> Subsystem3/9(r_leak_in)
  Subsystem2/8(r_out) -> Subsystem3/8(r_in)
  Subsystem2/7(c_out) -> Subsystem3/7(c_in)
  Subsystem2/6(i_out) -> Subsystem3/6(i_in)
  Subsystem2/5(p_leak_out) -> Subsystem3/5(p_leak_in)
  Subsystem2/4(p_chg_out) -> Subsystem3/4(p_chg_in)
  Subsystem2/3(i_leak_out) -> Subsystem3/3(i_leak_in)
  Subsystem2/2(v_cap_out) -> Subsystem3/2(v_cap_in)
  Subsystem2/1(v_r_out) -> Subsystem3/1(v_r_in)
  Subsystem1/10(l_out) -> Subsystem2/10(l_in)
  Subsystem1/9(r_leak_out) -> Subsystem2/9(r_leak_in)
  Subsystem1/8(r_out) -> Subsystem2/8(r_in)
  Subsystem1/7(c_out) -> Subsystem2/7(c_in)
  Subsystem1/6(i_out) -> Subsystem2/6(i_in)
  Subsystem1/5(p_leak_out) -> Subsystem2/5(p_leak_in)
  Subsystem1/4(p_chg_out) -> Subsystem2/4(p_chg_in)
  Subsystem1/3(i_leak_out) -> Subsystem2/3(i_leak_in)
  Subsystem1/2(v_cap_out) -> Subsystem2/2(v_cap_in)
  Subsystem1/1(v_r_out) -> Subsystem2/1(v_r_in)
  Subsystem5/10(l_out) -> Subsystem1/10(l_in)
  Subsystem5/9(r_leak_out) -> Subsystem1/9(r_leak_in)
  Subsystem5/8(r_out) -> Subsystem1/8(r_in)
  Subsystem5/7(c_out) -> Subsystem1/7(c_in)
  Subsystem5/6(i_out) -> Subsystem1/6(i_in)
  Subsystem5/5(p_leak_out) -> Subsystem1/5(p_leak_in)
  Subsystem5/4(p_chg_out) -> Subsystem1/4(p_chg_in)
  Subsystem5/3(i_leak_out) -> Subsystem1/3(i_leak_in)
  Subsystem5/2(v_cap_out) -> Subsystem1/2(v_cap_in)
  Subsystem5/1(v_r_out) -> Subsystem1/1(v_r_in)
  In10/1 -> Subsystem5/10(l_in)
  In9/1 -> Subsystem5/9(r_leak_in)
  In8/1 -> Subsystem5/8(r_in)
  In7/1 -> Subsystem5/7(c_in)
  In6/1 -> Subsystem5/6(i_in)
  In5/1 -> Subsystem5/5(p_leak_in)
  In4/1 -> Subsystem5/4(p_chg_in)
  In3/1 -> Subsystem5/3(i_leak_in)
  In2/1 -> Subsystem5/2(v_cap_in)
  In1/1 -> Subsystem5/1(v_r_in)
  connections:
  Subsystem6/RConn2 -- Conn4/RConn1
  Subsystem6/RConn1 -- Conn2/RConn1
  Subsystem6/LConn2 -- Subsystem4/RConn2
  Subsystem6/LConn1 -- Subsystem4/RConn1
  Subsystem4/LConn2 -- Subsystem3/RConn2
  Subsystem4/LConn1 -- Subsystem3/RConn1
  Subsystem3/LConn2 -- Subsystem2/RConn2
  Subsystem3/LConn1 -- Subsystem2/RConn1
  Subsystem2/LConn2 -- Subsystem1/RConn2
  Subsystem2/LConn1 -- Subsystem1/RConn1
  Subsystem1/LConn2 -- Subsystem5/RConn2
  Subsystem1/LConn1 -- Subsystem5/RConn1
  Conn3/RConn1 -- Subsystem5/LConn2
  Conn1/RConn1 -- Subsystem5/LConn1

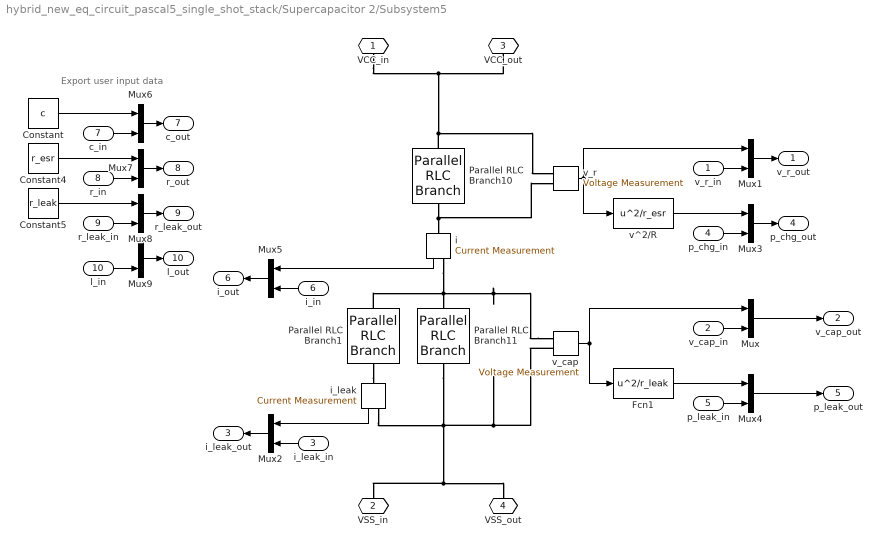
== system hybrid_new_eq_circuit_pascal5_single_shot_stack/Supercapacitor 2/Subsystem5 ==
  note: Export user input data
  v_r_in : Inport
  v_cap_in : Inport  Port=2
  i_leak_in : Inport  Port=3
  p_chg_in : Inport  Port=4
  p_leak_in : Inport  Port=5
  i_in : Inport  Port=6
  c_in : Inport  Port=7
  r_in : Inport  Port=8
  r_leak_in : Inport  Port=9
  l_in : Inport  Port=10
  Constant : Constant  Value=c
  Constant4 : Constant  Value=r_esr
  Constant5 : Constant  Value=r_leak
  Fcn1 : Fcn  Expr=u^2/r_leak
  Mux{,1..9} (10 alike) : Mux  Inputs=2
  Parallel RLC Branch1 : powerlib/Elements/Parallel RLC Branch  LConnTagsString=a  RConnTagsString=__new0  BranchType=R  Resistance=r_esr  Inductance=1e-3  SetiL0=off  InitialCurrent=0  Capacitance=1e-6  Setx0=off  InitialVoltage=0  Measurements=None
      settings: SourceProductName=Simscape Electrical
  Parallel RLC Branch10 : powerlib/Elements/Parallel RLC Branch  LConnTagsString=a  RConnTagsString=__new0  BranchType=R  Resistance=r_esr  Inductance=1e-3  SetiL0=off  InitialCurrent=0  Capacitance=1e-6  Setx0=off  InitialVoltage=0  Measurements=None
      settings: SourceProductName=Simscape Electrical
  Parallel RLC Branch11 : powerlib/Elements/Parallel RLC Branch  LConnTagsString=a  RConnTagsString=__new0  BranchType=C  Resistance=1  Inductance=1e-3  SetiL0=off  InitialCurrent=0  Capacitance=c  Setx0=on  InitialVoltage=v_init  Measurements=None
      settings: SourceProductName=Simscape Electrical
  i : powerlib/Measurements/Current Measurement  PhasorSimulation=off  OutputType=Complex  PSBequivalent=0
      settings: SourceProductName=Simscape Electrical
  i_leak : powerlib/Measurements/Current Measurement  PhasorSimulation=off  OutputType=Complex  PSBequivalent=0
      settings: SourceProductName=Simscape Electrical
  v^2/R : Fcn  Expr=u^2/r_esr
  v_cap : powerlib/Measurements/Voltage Measurement  PhasorSimulation=off  OutputType=Complex  PSBequivalent=0
      settings: SourceProductName=Simscape Electrical
  v_r : powerlib/Measurements/Voltage Measurement  PhasorSimulation=off  OutputType=Complex  PSBequivalent=0
      settings: SourceProductName=Simscape Electrical
  VCC_in : PMIOPort  Side=Left
  VSS_in : PMIOPort  Port=2  Side=Left
  VCC_out : PMIOPort  Tag=PMCPort  Port=3  Side=Right
  VSS_out : PMIOPort  Tag=PMCPort  Port=4  Side=Right
  v_r_out : Outport
  v_cap_out : Outport  Port=2
  i_leak_out : Outport  Port=3
  p_chg_out : Outport  Port=4
  p_leak_out : Outport  Port=5
  i_out : Outport  Port=6
  c_out : Outport  Port=7
  r_out : Outport  Port=8
  r_leak_out : Outport  Port=9
  l_out : Outport  Port=10
  wires:
  Fcn1/1 -> Mux4/1
  v_cap/1 -> Mux/1, Fcn1/1
  v_cap_in/1 -> Mux/2
  Mux/1 -> v_cap_out/1
  Mux4/1 -> p_leak_out/1
  p_leak_in/1 -> Mux4/2
  i_in/1 -> Mux5/2
  Mux5/1 -> i_out/1
  i/1 -> Mux5/1
  i_leak_in/1 -> Mux2/2
  Mux2/1 -> i_leak_out/1
  v^2/R/1 -> Mux3/1
  Mux1/1 -> v_r_out/1
  v_r_in/1 -> Mux1/2
  Mux3/1 -> p_chg_out/1
  p_chg_in/1 -> Mux3/2
  r_in/1 -> Mux7/2
  r_leak_in/1 -> Mux8/2
  l_in/1 -> Mux9/2
  c_in/1 -> Mux6/2
  ? -> Mux9/1
  Constant5/1 -> Mux8/1
  Constant4/1 -> Mux7/1
  Constant/1 -> Mux6/1
  Mux9/1 -> l_out/1
  Mux8/1 -> r_leak_out/1
  Mux7/1 -> r_out/1
  Mux6/1 -> c_out/1
  v_r/1 -> v^2/R/1, Mux1/1
  i_leak/1 -> Mux2/1
  connections:
  Parallel RLC Branch10/RConn1 -- i/LConn1 -- v_r/LConn2
  VCC_in/RConn1 -- Parallel RLC Branch10/LConn1 -- v_r/LConn1 -- VCC_out/RConn1
  v_cap/LConn1 -- Parallel RLC Branch11/LConn1 -- i/RConn1 -- Parallel RLC Branch1/LConn1
  v_cap/LConn2 -- Parallel RLC Branch11/RConn1 -- i_leak/RConn1 -- VSS_in/RConn1 -- VSS_out/RConn1
  Parallel RLC Branch1/RConn1 -- i_leak/LConn1
